simulink model "Counter"  (R2021a)
settings: Solver=VariableStepAuto  StartTime=0.0  StopTime=10.0  RelTol=1e-3
settings Model: Creator=Moamen_Hamed  LastModifiedBy=Moamen_Hamed

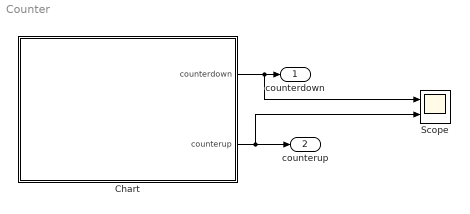
== system Counter ==
  Chart : Stateflow chart  TreatAsAtomicUnit=on
  Scope : Scope  NumInputPorts=2
  counterdown : Outport
  counterup : Outport  Port=2
  wires:
  Chart/1(counterdown) -> Scope/1, counterdown/1
  Chart/2(counterup) -> Scope/2, counterup/1

== stateflow chart Counter/Chart ==
  state init
    entry:
    counterup = 0;
    counterdown = 10;
  state Counter
    entry:
    counterup = counterup + 1;
    counterdown = counterdown - 1;
  (default) -> init
  init -> Counter
  Counter -> Counter [order 2] : [after(1,tick)]
  Counter -> Counter [order 1] : [counterup == 10]{counterup = -1;counterdown=11;}
  data: counter local; counterdown output; counterup output
